simulink model "spaceShuttleOriginal"  (R2017b)
settings: Solver=FixedStepAuto  StartTime=0.0  StopTime=300  FixedStep=0.08  RelTol=1e-3
undefined symbols (not defined in the file or in its folder): ATTITUDE_ESTIMATE, ATTITUDE_INCREMENT, AUTO_MANUAL_SWITCH, BYPASS, COUNTER, CURRENT_ATTITUDE, DESIRED_ATTITUDE, DESIRED_RATE, INIT_AUTO_MANEUVER, INIT_JET_SELECT, INIT_STATE_ERROR, MANEUVER_HOLD_SW, PRIMARY_JET_COMMAND, RATE_ESTIMATE, UNDESIRED_ACCELERATION_ESTIMATE, VERNIER_JET_COMMAND
libraries: sharedtransform x5, aerolibutil x4, realtime_pacer_lib x1
(part 3 of 3)

== matlab function spaceShuttleOriginal/Auto // Manual Maneuver/If AUTO/IF COUNTER=0/AUTO MANEUVER MODULE/MATLAB Function1 ==
  data: q input; U output
function U = getAxis(q)
y = [0;0;0];
y(1) = q(2);
y(2) = q(3);
y(3) = q(4);
if norm(y) == 0
    U = [1;0;0];
else
    U = -y/norm(y);
end

== matlab function spaceShuttleOriginal/Auto // Manual Maneuver/If AUTO/IF COUNTER=0/AUTO MANEUVER MODULE/MATLAB Function ==
  data: q input; theta output
function theta = getAngle(q)
y = [0;0;0];
y(1) = q(2);
y(2) = q(3);
y(3) = q(4);
theta = 2*asin(sqrt( q(2)^2 + q(3)^2 + q(4)^2 ) );

== matlab function spaceShuttleOriginal/Call Jet Select/VERNIER JETS/MATLAB Function ==
  data: vernierJetCommand output
function vernierJetCommand  = vernier_jet_logic()
vernierJetCommand = zeros(6,1);

== matlab function spaceShuttleOriginal/Call Phase Plane/Get Rotation Pitch/MATLAB Function ==
  data: n input; S output; vernier_sw input; undesired_acc input; DB input; attitude_error input; rate_error input; rotationCommandn input; rateLimit input
function S = region_limit ( n, vernier_sw,undesired_acc, DB, attitude_error,...
                                            rate_error, rotationCommandn, rateLimit)

if vernier_sw == 1
    data_alpha_c = [0.64;0.72;0.48];
    data_omega_min = [0.64;0.072;0.048];
else
    data_alpha_c =  [0.0152;0.0104;0.0112];
    data_omega_min = [0.00152;0.00104;0.00112];
end

alpha_c = data_alpha_c(n);
omega_min = data_omega_min(n);
alpha_d = undesired_acc(n);

alpha_c_p = alpha_c - sign(rate_error(n))*alpha_d;
S1 = DB - rate_error(n)^2/(2*alpha_c_p);
S7 = -S1;

if abs(rotationCommandn(n)) == 1
    C = 1;
else
    C = 1.25;
end
S8 = C*rate_error(n)^2/(2*alpha_c_p) + 1.2*DB;
S2 = -1*S8;
S3 = rateLimit;
S9 = -rateLimit;
S4 = 0.8*rateLimit;
S10 = -1*S4;
if vernier_sw == 0
    S5 = 0.5*rateLimit;
else
    S5 = rateLimit - 2*omega_min;
end
S11 = -1*S5;
S12 = rate_error(n)^2/(2*alpha_c_p) + DB;
S6 = -1*S12;
K = sign(alpha_d) * attitude_error(n);

if  K <= -0.5*DB
    S13 = 0;
else
    S13 = -sign(alpha_d) * (sqrt((K+0.5*DB)*2*abs(alpha_d))-omega_min);
end

if S13 * alpha_d > 0
    S13 = 0;
end

if abs(S13) > rateLimit - omega_min 
    S13 = sign(alpha_d) * (omega_min - rateLimit);
end

S = [S1 S2 S3 S4 S5 S6 S7 S8 S9 S10 S11 S12 S13];

end

== matlab function spaceShuttleOriginal/Call Phase Plane/Get Rotation Yaw/MATLAB Function ==
  data: n input; S output; vernier_sw input; undesired_acc input; DB input; attitude_error input; rate_error input; rotationCommandn input; rateLimit input
function S = region_limit ( n, vernier_sw,undesired_acc, DB, attitude_error,...
                                            rate_error, rotationCommandn, rateLimit)

if vernier_sw == 1
    data_alpha_c = [0.64;0.72;0.48];
    data_omega_min = [0.64;0.072;0.048];
else
    data_alpha_c =  [0.0152;0.0104;0.0112];
    data_omega_min = [0.00152;0.00104;0.00112];
end

alpha_c = data_alpha_c(n);
omega_min = data_omega_min(n);
alpha_d = undesired_acc(n);

alpha_c_p = alpha_c - sign(rate_error(n))*alpha_d;
S1 = DB - rate_error(n)^2/(2*alpha_c_p);
S7 = -S1;

if abs(rotationCommandn(n)) == 1
    C = 1;
else
    C = 1.25;
end
S8 = C*rate_error(n)^2/(2*alpha_c_p) + 1.2*DB;
S2 = -1*S8;
S3 = rateLimit;
S9 = -rateLimit;
S4 = 0.8*rateLimit;
S10 = -1*S4;
if vernier_sw == 0
    S5 = 0.5*rateLimit;
else
    S5 = rateLimit - 2*omega_min;
end
S11 = -1*S5;
S12 = rate_error(n)^2/(2*alpha_c_p) + DB;
S6 = -1*S12;
K = sign(alpha_d) * attitude_error(n);

if  K <= -0.5*DB
    S13 = 0;
else
    S13 = -sign(alpha_d) * (sqrt((K+0.5*DB)*2*abs(alpha_d))-omega_min);
end

if S13 * alpha_d > 0
    S13 = 0;
end

if abs(S13) > rateLimit - omega_min 
    S13 = sign(alpha_d) * (omega_min - rateLimit);
end

S = [S1 S2 S3 S4 S5 S6 S7 S8 S9 S10 S11 S12 S13];

end

== matlab function spaceShuttleOriginal/Call Phase Plane/Get Rotation Pitch/MATLAB Function1 ==
  data: n input; S input; index output; theta_e input; we input; undesired_acc input
function index = affectation_region(n, S, theta_e, we, undesired_acc)

attitude_error = theta_e(n);
rate_error = we(n);
alpha_d = undesired_acc(n);
S1 = S(1);
S2 = S(2);
S3 = S(3);
S4 = S(3);
S5 = S(5);
S6 = S(6);
S7 = S(7);
S8 = S(8);
S9 = S(9);
S10 = S(10);
S11 = S(11);
S12 = S(12);
S13 = S(13);

index = 0;

if ( (attitude_error > S1 && rate_error > 0) || ...
     (attitude_error < S8 && rate_error > S11 ) ||  ...
     (rate_error > S3  )  )
    index = 1;
end


if ( (attitude_error < S7 && rate_error <= 0) || ...
     (attitude_error < S2 && rate_error > S5 ) ||  ...
     (rate_error < S9  )  )
    index = 5;
end

if ( attitude_error < S2 )
    if (S4 <= rate_error) && (rate_error <= S3)
        index = 2;
    end
    if (S5 <= rate_error) && (rate_error < S4)
        index = 3;
    end
end

if ( attitude_error > S8 )
    if (S10 >= rate_error) && (rate_error >= S9)
        index = 6;
    end
    if (S11 >= rate_error) && (rate_error > S10)
        index = 7;
    end
end

if ( alpha_d >= 0 )
    if ( ((S6 <= attitude_error) && (attitude_error <= S1) &&  (0 <= rate_error) &&  (rate_error <= S3) ) || ...
           ( (S13 <= rate_error) && (rate_error < 0) && (attitude_error <= S8 ) ) )
        index = 4;
    end
    if ( (S12 >= attitude_error) && (attitude_error >= S7) &&  (S13 > rate_error) &&  (rate_error >= S9) )
        index = 8;
    end
else
    if ( (S6 <= attitude_error) && (attitude_error <= S1) &&  (S13 < rate_error) &&  (rate_error <= S3) )
        index = 4;
    end 
    if ( ((S12 >= attitude_error) && (attitude_error >= S7) &&  (0 >= rate_error) &&  (rate_error >= S9) ) || ...
           ( (S13 >= rate_error) && (rate_error > 0) && (attitude_error >= S2 ) ) )
        index = 8;
    end
end

if ( ((S2 <= attitude_error) && (attitude_error < S6) &&  (S13 < rate_error) &&  (rate_error <= S3) ) || ...
           ( (S8 >= attitude_error) && (attitude_error > S12) && (S13 > rate_error) &&  (rate_error >= S9) ) )
        index = 9;
end

end

== matlab function spaceShuttleOriginal/Attitude Processing/SECOND_PASS == 1/ATTITUDE PROCESSOR/MATLAB Function2 ==
  data: u input; x output
function x = fcn2(u)
x = zeros(3,1);
theta = 2* asin(sqrt(u(2)^2 + u(3)^2 + u(4)^2));
a = sqrt(u(2)^2 + u(3)^2 + u(4)^2);
if a == 0
    x = [0;0;0];
else
    x(1) = -1*theta * u(2) / a;
    x(2) = -1*theta * u(3) / a;
    x(3) = -1*theta * u(4) / a;
end
end

== matlab function spaceShuttleOriginal/Attitude Processing/SECOND_PASS == 1/ATTITUDE PROCESSOR/MATLAB Function3 ==
  data: u input; x output
function x = fcn_test(u)
x = rotm2eul(u);
end

== matlab function spaceShuttleOriginal/Call Phase Plane/Get Rotation Yaw/MATLAB Function1 ==
  data: n input; S input; index output; theta_e input; we input; undesired_acc input
function index = affectation_region(n, S, theta_e, we, undesired_acc)

attitude_error = theta_e(n);
rate_error = we(n);
alpha_d = undesired_acc(n);
S1 = S(1);
S2 = S(2);
S3 = S(3);
S4 = S(3);
S5 = S(5);
S6 = S(6);
S7 = S(7);
S8 = S(8);
S9 = S(9);
S10 = S(10);
S11 = S(11);
S12 = S(12);
S13 = S(13);

index = 0;

if ( (attitude_error > S1 && rate_error > 0) || ...
     (attitude_error < S8 && rate_error > S11 ) ||  ...
     (rate_error > S3  )  )
    index = 1;
end


if ( (attitude_error < S7 && rate_error <= 0) || ...
     (attitude_error < S2 && rate_error > S5 ) ||  ...
     (rate_error < S9  )  )
    index = 5;
end

if ( attitude_error < S2 )
    if (S4 <= rate_error) && (rate_error <= S3)
        index = 2;
    end
    if (S5 <= rate_error) && (rate_error < S4)
        index = 3;
    end
end

if ( attitude_error > S8 )
    if (S10 >= rate_error) && (rate_error >= S9)
        index = 6;
    end
    if (S11 >= rate_error) && (rate_error > S10)
        index = 7;
    end
end

if ( alpha_d >= 0 )
    if ( ((S6 <= attitude_error) && (attitude_error <= S1) &&  (0 <= rate_error) &&  (rate_error <= S3) ) || ...
           ( (S13 <= rate_error) && (rate_error < 0) && (attitude_error <= S8 ) ) )
        index = 4;
    end
    if ( (S12 >= attitude_error) && (attitude_error >= S7) &&  (S13 > rate_error) &&  (rate_error >= S9) )
        index = 8;
    end
else
    if ( (S6 <= attitude_error) && (attitude_error <= S1) &&  (S13 < rate_error) &&  (rate_error <= S3) )
        index = 4;
    end 
    if ( ((S12 >= attitude_error) && (attitude_error >= S7) &&  (0 >= rate_error) &&  (rate_error >= S9) ) || ...
           ( (S13 >= rate_error) && (rate_error > 0) && (attitude_error >= S2 ) ) )
        index = 8;
    end
end

if ( ((S2 <= attitude_error) && (attitude_error < S6) &&  (S13 < rate_error) &&  (rate_error <= S3) ) || ...
           ( (S8 >= attitude_error) && (attitude_error > S12) && (S13 > rate_error) &&  (rate_error >= S9) ) )
        index = 9;
end

end

== matlab function spaceShuttleOriginal/Call Phase Plane/Get Rotation Yaw/MATLAB Function2 ==
  data: n input; index input; S input; vernier_sw input; command output; BYPASS input; RC input; rate_error input; rateLimit input; forceFire input
function command = phase_plane(n, index, S, vernier_sw, BYPASS, RC, rate_error, rateLimit, forceFire)
rotationCommand = RC(n);
we = rate_error(n);
forceFire_n = forceFire(n);
bypass_n = BYPASS(n);


command = -100;


if (bypass_n == 0)
    if (index == 1)        
        command = -1;    
    end
    if (index == 5)        
        command = 1;     
    end
    if (index == 2)   || (index == 3) || (index == 6) || (index == 7)      
        if vernier_sw == 1
            command =0;
        else
            if ( ( (index == 2) &&  (rotationCommand ~= 1) ) || ...
                ( (index == 3) &&  (rotationCommand ~= 1) )  )
                command  = 3.2-4*we/(rateLimit);
            end
            if ( ( (index == 6) &&  (rotationCommand ~= 1) ) || ...
                ( (index == 7) &&  (rotationCommand ~= 1) )  )
                command  = 3.2-4*we/(rateLimit);
            end
        end
            
    end
    if ((index == 4) && rotationCommand ~= -1  )
        if forceFire_n == 1
            command = -1;
        else
            command = 0.8*(S(13)-we) / (rateLimit - S(13));
        end
    end
    
     if ((index == 8) && rotationCommand ~= -1  )
        if forceFire_n == 1
            command = 1;
        else
            command = 0.8*(S(13)-we) / (rateLimit + S(13));
        end        
    end   
        
     if (index == 9) 
         command = 0.8 * (S(13) - we) * (rateLimit - sign(we)*S(13));             
     end  
end
end

== matlab function spaceShuttleOriginal/Call Phase Plane/Get Rotation Pitch/MATLAB Function2 ==
  data: n input; index input; S input; vernier_sw input; command output; BYPASS input; RC input; rate_error input; rateLimit input; forceFire input
function command = phase_plane(n, index, S, vernier_sw, BYPASS, RC, rate_error, rateLimit, forceFire)
rotationCommand = RC(n);
we = rate_error(n);
forceFire_n = forceFire(n);
bypass_n = BYPASS(n);


command = -100;


if (bypass_n == 0)
    if (index == 1)        
        command = -1;    
    end
    if (index == 5)        
        command = 1;     
    end
    if (index == 2)   || (index == 3) || (index == 6) || (index == 7)      
        if vernier_sw == 1
            command =0;
        else
            if ( ( (index == 2) &&  (rotationCommand ~= 1) ) || ...
                ( (index == 3) &&  (rotationCommand ~= 1) )  )
                command  = 3.2-4*we/(rateLimit);
            end
            if ( ( (index == 6) &&  (rotationCommand ~= 1) ) || ...
                ( (index == 7) &&  (rotationCommand ~= 1) )  )
                command  = 3.2-4*we/(rateLimit);
            end
        end
            
    end
    if ((index == 4) && rotationCommand ~= -1  )
        if forceFire_n == 1
            command = -1;
        else
            command = 0.8*(S(13)-we) / (rateLimit - S(13));
        end
    end
    
     if ((index == 8) && rotationCommand ~= -1  )
        if forceFire_n == 1
            command = 1;
        else
            command = 0.8*(S(13)-we) / (rateLimit + S(13));
        end        
    end   
        
     if (index == 9) 
         command = 0.8 * (S(13) - we) * (rateLimit - sign(we)*S(13));             
     end  
end
end

== matlab function spaceShuttleOriginal/Call Phase Plane/Get Rotation Roll/MATLAB Function ==
  data: n input; S output; vernier_sw input; undesired_acc input; DB input; attitude_error input; rate_error input; rotationCommandn input; rateLimit input
function S = region_limit ( n, vernier_sw,undesired_acc, DB, attitude_error,...
                                            rate_error, rotationCommandn, rateLimit)

if vernier_sw == 1
    data_alpha_c = [0.64;0.72;0.48];
    data_omega_min = [0.64;0.072;0.048];
else
    data_alpha_c =  [0.0152;0.0104;0.0112];
    data_omega_min = [0.00152;0.00104;0.00112];
end

alpha_c = data_alpha_c(n);
omega_min = data_omega_min(n);
alpha_d = undesired_acc(n);

alpha_c_p = alpha_c - sign(rate_error(n))*alpha_d;
S1 = DB - rate_error(n)^2/(2*alpha_c_p);
S7 = -S1;

if abs(rotationCommandn(n)) == 1
    C = 1;
else
    C = 1.25;
end
S8 = C*rate_error(n)^2/(2*alpha_c_p) + 1.2*DB;
S2 = -1*S8;
S3 = rateLimit;
S9 = -rateLimit;
S4 = 0.8*rateLimit;
S10 = -1*S4;
if vernier_sw == 0
    S5 = 0.5*rateLimit;
else
    S5 = rateLimit - 2*omega_min;
end
S11 = -1*S5;
S12 = rate_error(n)^2/(2*alpha_c_p) + DB;
S6 = -1*S12;
K = sign(alpha_d) * attitude_error(n);

if  K <= -0.5*DB
    S13 = 0;
else
    S13 = -sign(alpha_d) * (sqrt((K+0.5*DB)*2*abs(alpha_d))-omega_min);
end

if S13 * alpha_d > 0
    S13 = 0;
end

if abs(S13) > rateLimit - omega_min 
    S13 = sign(alpha_d) * (omega_min - rateLimit);
end

S = [S1 S2 S3 S4 S5 S6 S7 S8 S9 S10 S11 S12 S13];

end

== matlab function spaceShuttleOriginal/Call Phase Plane/Get Rotation Roll/MATLAB Function1 ==
  data: n input; S input; index output; theta_e input; we input; undesired_acc input
function index = affectation_region(n, S, theta_e, we, undesired_acc)

attitude_error = theta_e(n);
rate_error = we(n);
alpha_d = undesired_acc(n);
S1 = S(1);
S2 = S(2);
S3 = S(3);
S4 = S(3);
S5 = S(5);
S6 = S(6);
S7 = S(7);
S8 = S(8);
S9 = S(9);
S10 = S(10);
S11 = S(11);
S12 = S(12);
S13 = S(13);

index = 0;

if ( (attitude_error > S1 && rate_error > 0) || ...
     (attitude_error < S8 && rate_error > S11 ) ||  ...
     (rate_error > S3  )  )
    index = 1;
end


if ( (attitude_error < S7 && rate_error <= 0) || ...
     (attitude_error < S2 && rate_error > S5 ) ||  ...
     (rate_error < S9  )  )
    index = 5;
end

if ( attitude_error < S2 )
    if (S4 <= rate_error) && (rate_error <= S3)
        index = 2;
    end
    if (S5 <= rate_error) && (rate_error < S4)
        index = 3;
    end
end

if ( attitude_error > S8 )
    if (S10 >= rate_error) && (rate_error >= S9)
        index = 6;
    end
    if (S11 >= rate_error) && (rate_error > S10)
        index = 7;
    end
end

if ( alpha_d >= 0 )
    if ( ((S6 <= attitude_error) && (attitude_error <= S1) &&  (0 <= rate_error) &&  (rate_error <= S3) ) || ...
           ( (S13 <= rate_error) && (rate_error < 0) && (attitude_error <= S8 ) ) )
        index = 4;
    end
    if ( (S12 >= attitude_error) && (attitude_error >= S7) &&  (S13 > rate_error) &&  (rate_error >= S9) )
        index = 8;
    end
else
    if ( (S6 <= attitude_error) && (attitude_error <= S1) &&  (S13 < rate_error) &&  (rate_error <= S3) )
        index = 4;
    end 
    if ( ((S12 >= attitude_error) && (attitude_error >= S7) &&  (0 >= rate_error) &&  (rate_error >= S9) ) || ...
           ( (S13 >= rate_error) && (rate_error > 0) && (attitude_error >= S2 ) ) )
        index = 8;
    end
end

if ( ((S2 <= attitude_error) && (attitude_error < S6) &&  (S13 < rate_error) &&  (rate_error <= S3) ) || ...
           ( (S8 >= attitude_error) && (attitude_error > S12) && (S13 > rate_error) &&  (rate_error >= S9) ) )
        index = 9;
end

end

== matlab function spaceShuttleOriginal/Call Phase Plane/Get Rotation Roll/MATLAB Function2 ==
  data: n input; index input; S input; vernier_sw input; command output; BYPASS input; RC input; rate_error input; rateLimit input; forceFire input
function command = phase_plane(n, index, S, vernier_sw, BYPASS, RC, rate_error, rateLimit, forceFire)
rotationCommand = RC(n);
we = rate_error(n);
forceFire_n = forceFire(n);
bypass_n = BYPASS(n);


command = -100;


if (bypass_n == 0)
    if (index == 1)        
        command = -1;    
    end
    if (index == 5)        
        command = 1;     
    end
    if (index == 2)   || (index == 3) || (index == 6) || (index == 7)      
        if vernier_sw == 1
            command =0;
        else
            if ( ( (index == 2) &&  (rotationCommand ~= 1) ) || ...
                ( (index == 3) &&  (rotationCommand ~= 1) )  )
                command  = 3.2-4*we/(rateLimit);
            end
            if ( ( (index == 6) &&  (rotationCommand ~= 1) ) || ...
                ( (index == 7) &&  (rotationCommand ~= 1) )  )
                command  = 3.2-4*we/(rateLimit);  
            end
        end
            
    end
    if ((index == 4) && rotationCommand ~= -1  )
        if forceFire_n == 1
            command = -1;
        else
            command = 0.8*(S(13)-we) / (rateLimit - S(13));
        end
    end
    
     if ((index == 8) && rotationCommand ~= -1  )
        if forceFire_n == 1
            command = 1;
        else
            command = 0.8*(S(13)-we) / (rateLimit + S(13));
        end        
    end   
        
     if (index == 9) 
         command = 0.8 * (S(13) - we) * (rateLimit - sign(we)*S(13));             
     end  
end
end

== matlab function spaceShuttleOriginal/Call Jet Select/PRIMARY JETS/MATLAB Function ==
  data: compensationCommand input; rotationCommand input; primaryJetCommand output; PITCH_HI_LOW_SW input; NO_PLUS_Z_JETS input; PITCH_TAIL_NOSE_SW input; YAW_HI_LOW_SW input; YAW_TAIL_NOSE_SW input
function primaryJetCommand  = primary_jet_logic(compensationCommand, rotationCommand, PITCH_HI_LOW_SW, ...
    NO_PLUS_Z_JETS, PITCH_TAIL_NOSE_SW, YAW_HI_LOW_SW, YAW_TAIL_NOSE_SW)

bitCommand = zeros(6,1);
primaryJetCommand = zeros(11,1);

for i=1:3
   j = 2*i;
   if abs(rotationCommand(i)) == 1 || abs(compensationCommand(i)) == 1
       bitCommand(j) = 1;
   else
       bitCommand(j) = 0;
   end
   if rotationCommand(i) == -1 || ( rotationCommand(i) ~= 1 && compensationCommand(i) == -1 )
       bitCommand(j-1) = 1;
   else
       bitCommand(j-1) = 0;
   end   
end
HI_PITCH = PITCH_HI_LOW_SW || NO_PLUS_Z_JETS;
NOSE_PITCH = not(bitCommand(2) || HI_PITCH || PITCH_TAIL_NOSE_SW);
TAIL_PITCH = not( HI_PITCH || NOSE_PITCH );
C1 = not(TAIL_PITCH);
primaryJetCommand(1) = bitCommand(3) && bitCommand(4) && C1 && not(NO_PLUS_Z_JETS);
primaryJetCommand(2) = not(bitCommand(3)) && bitCommand(4) && C1;
primaryJetCommand(3) = primaryJetCommand(2);
C1 = not(bitCommand(3)) || not(bitCommand(4)) ;
C2 = not(bitCommand(2)) && not(bitCommand(3)) && bitCommand(4);
C3 = not(NOSE_PITCH) && not(NO_PLUS_Z_JETS);
primaryJetCommand(4) = ((bitCommand(1) && bitCommand(2) && C1) || C2 ) && C3;
primaryJetCommand(5) = ((not(bitCommand(1)) && bitCommand(2) && C1 ) || C2 ) && C3;
C1 = NO_PLUS_Z_JETS || bitCommand(3) || not(bitCommand(4));
C2 = not(bitCommand(2)) && bitCommand(3) && bitCommand(4);
primaryJetCommand(6) = (( not(bitCommand(1)) && bitCommand(2) && C1) || C2 ) && not(NOSE_PITCH);
primaryJetCommand(7) = (( bitCommand(1) && bitCommand(2) && C1) || C2) && not(NOSE_PITCH);
C1 = ( YAW_HI_LOW_SW || not(YAW_TAIL_NOSE_SW) )  && bitCommand(6);
primaryJetCommand(8) = not(bitCommand(5)) && C1;
primaryJetCommand(9) = bitCommand(5) && C1;
C1 = ( YAW_HI_LOW_SW || YAW_TAIL_NOSE_SW )  && bitCommand(6);
primaryJetCommand(10) = bitCommand(5) && C1;
primaryJetCommand(11) = not(bitCommand(5)) && C1;

== matlab function spaceShuttleOriginal/Subsystem/MATLAB Function ==
  data: JetCommand input; delta_omega output
function delta_omega = get_delta_omega(JetCommand)

delta_omega = [0;0;0];

matrix_delta_omega_jet = [   0       -0.03389  0       ;...  %1
                            -0.01775  0.02513 -0.02364 ;...  %2
                             0.01778  0.02514  0.02363 ;...  %3
                            -0.03573  0.01901 -0.00293 ;...  %4
                             0.03607  0.01904  0.00294 ;...  %5
                             0.02849 -0.01281 -0.00458 ;...  %6
                            -0.02876 -0.01284  0.00457 ;...  %7
                             0.00547 -0.00037  0.03194 ;...  %8
                            -0.00547 -0.00036 -0.03194 ;...  %9
                            0.02112   0       -0.01763 ;...  %10 
                           -0.02113   0        0.01763 ;...  %11
                           -0.0004152  0.0007067 -0.0006653  ;...    %12
                            0.0004162  0.0007069  0.0006652  ;...    %13
                           -0.0006727 -0.0000146  0.0005203  ;...    %14
                            0.0006724 -0.0000138 -0.0005203  ;...    %15
                           -0.0005994 -0.0003125 -0.0000201  ;...    %16
                            0.0005942 -0.0003120 0.0000200] ;        %17
                       
for i=1:length(JetCommand)
    if (JetCommand(i) == 1)
        delta_omega = delta_omega + matrix_delta_omega_jet(i,:)';
    end
end

== matlab function spaceShuttleOriginal/Attitude Processing/SECOND_PASS == 1/State Estimator Part I/MATLAB Function2 ==
  data: u input; x output
function x = fcn2(u)
x = zeros(3,1);
theta = 2* asin(sqrt(u(2)^2 + u(3)^2 + u(4)^2));
a = sqrt(u(2)^2 + u(3)^2 + u(4)^2);
if a == 0
    x = [0;0;0];
else
    x(1) = -1*theta * u(2) / a;
    x(2) = -1*theta * u(3) / a;
    x(3) = -1*theta * u(4) / a;
end
end
